simulink model "simpleInertiaModel"  (R2024a)
settings: Solver=ode23t  StartTime=0.0  StopTime=10  FixedStep=1e-3  MaxStep=0.01  RelTol=1e-3  AbsTol=1e-3  EnableMultiTasking=on
PreLoadFcn:
  | simpleInertiaModelParam
undefined symbols (not defined in the file): contact, objects, physics, ramp, X, Y, Z
libraries: sm_lib x47, fl_lib x33, nesl_utility x29
(part 1 of 2)
settings Model: Creator=lnicolet  LastModifiedBy=lnicolet
settings SolverCC: AutoScaleAbsTol=off  AlgebraicLoopSolver=TrustRegion  MaxZcPerStep=1
settings DataIOCC: LimitDataPoints=on  MaxDataPoints=10000  ReturnWorkspaceOutputsName=ssmInertia
settings OptimizationCC: ReuseModelBlockBuffer=off  LifeSpan=inf
settings DebuggingCC: UnconnectedInputMsg=warning  UnconnectedOutputMsg=warning  UnconnectedLineMsg=warning  AllowSymbolicDim=off  SubsystemReferenceDiagnosticForUnitTest=warning  SFUnexpectedBacktrackingDiag=warning  SFNoUnconditionalDefaultTransitionDiag=warning  SFExecutionAtInitializationDiag=none  ArithmeticOperatorsInVariantConditions=warning
settings ModelReferenceCC: EnableRefExpFcnMdlSchedulingChecks=on
settings SFSimCC: SimUseLocalCustomCode=off  CustomCodeUndefinedFunction=UseInterfaceOnly
settings RTWCC: RTWUseLocalCustomCode=off  GPUComputeCapability=3.5  DLArmComputeVersion=19.05
settings CodeAppCC: StateflowObjectComments=on
settings GRTTargetCC: TargetLangStandard=C89/C90 (ANSI)
settings ConfigComp: CovMetricSettings=dw  CovSaveCumulativeToWorkspaceVar=on  CovSaveSingleToWorkspaceVar=on  CovExternalEMLEnable=off  CovSFcnEnable=off
settings SimscapeCC: SimscapeLogType=all  SimscapeLogSimulationStatistics=on  SimscapeLogLimitData=off  SimscapeLogDataHistory=10000
settings ExplorerConfigSet: InternalSimMechanicsExplorerSettings="<ExplorerConfiguration><canonicalview>default</canonicalview><AnimationSetting><BasePlaybackSpeed>1.0</BasePlaybackSpeed><PlaybackSpeedFactor>1.0</PlaybackSpeedFactor></AnimationSetting><TilePanel><TileInfo><Tiles Columns=\"1\" Count=\"1\" Rows=\"1\"><Column Weight=\"1\"/><Row Weight=\"1\"/><Tile Height=\"1\" Width=\"1\" X=\"0\" Y=\"0\"/></Tiles></TileInfo><SceneInfo><SceneViewer><BGColor><R>0.60000002384185791</R><G>0.60000002384185791</G><B>0.60000002384185791</B></BGColor><Camera><DoPerspective>off</DoPerspective><Position><X>16.2073991208090149</X><Y>-6.20739939897376747</Y><Z>8.70739941654175098</Z></Position><Center><X>9.99999967767763209</X><Y>4.41576100129736915e-08</Y><Z>2.49999997341037261</Z></Center><Up><X>-0.408248290463863073</X><Y>0.408248290463863073</Y><Z>0.816496580927726145</Z></Up><ViewLimDist>1</ViewLimDist><YLim>7.56892333507537884</YLim><XLim>11.6046355697525012</XLim></Camera></SceneViewer></SceneInfo></TilePanel><MechEditorPanel><Cameras/><GfxPanelCameraMap/><VideoCreator><PlaybackSpeedRatio>1.0</PlaybackSpeedRatio><FrameRate>30</FrameRate><VideoFormat>Motion JPEG AVI</VideoFormat><FrameSize>auto</FrameSize></VideoCreator></MechEditorPanel></ExplorerConfiguration>"

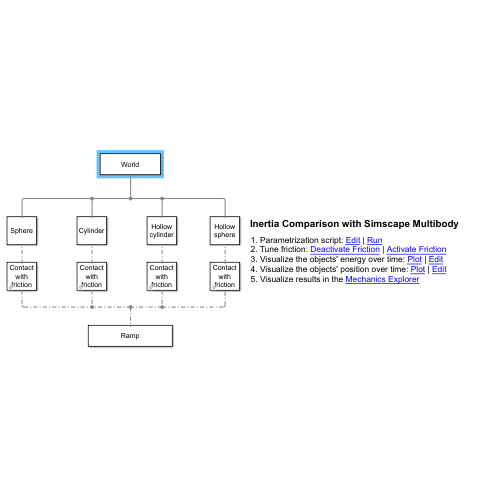
[thumbnail: Simulink's stored preview of the top-level diagram]
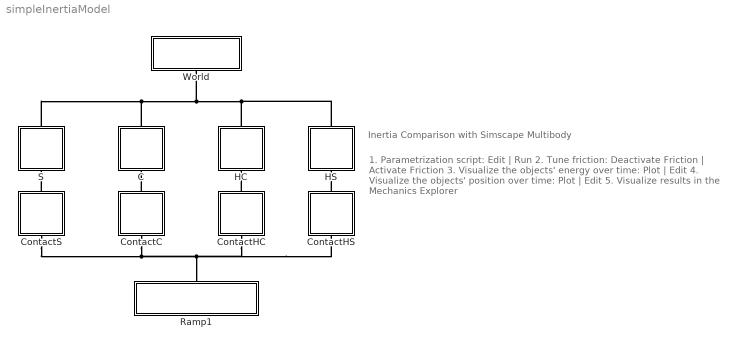
== system simpleInertiaModel ==
  note: 1. Parametrization script: Edit | Run
      | 2. Tune friction: Deactivate Friction | Activate Friction
      | 3. Visualize the objects' energy over time: Plot | Edit
      | 4. Visualize the objects' position over time: Plot | Edit
      | 5. Visualize results in the Mechanics Explorer
  note: Inertia Comparison with Simscape Multibody
  C : Subsystem
      mask Display: disp('Cylinder')
  ContactC : Subsystem  mask{c=contact.stiffness, d=contact.damping, tReg=contact.tansRegion, friction=Active, uS=contact.frictionStatic, uD=contact.frictionDynamic, v=contact.criticSpeed}
      mask prompts: c "Contact stiffness in N/m"; d "Contact damping in N/(m/s)"; tReg "Transition region in m"; friction "Contact Friction"; uS "Static friction coefficient"; uD "Dynamic friction coefficient"; v "Critical velocity in m/s"
      mask TypeOptions friction: Active | Inactive
      mask Callback friction:
      | ActiveChoice = get_param(gcb,'friction');
      | 
      |     switch ActiveChoice
      |         case 'Active'
      |             set_param([gcb,'/Ramp'],'FrictionType','SmoothStickSlip');
      |         case 'Inactive'
      |             set_param([gcb,'/Ramp'],'FrictionType','None');
      |     end
      mask DialogControl Container2 Prompt: Contact
      mask DialogControl Container3 Prompt: Friction
      mask Display:
      | ActiveChoice = get_param(gcb,'friction');
      | 
      | switch ActiveChoice
      |     case 'Active'
      |         disp('Contact\nwith\nfriction');
      |     case 'Inactive'
      |         disp('Contact\nwithout\nfriction');
      | end
  ContactHC : Subsystem  mask{c=contact.stiffness, d=contact.damping, tReg=contact.tansRegion, friction=Active, uS=contact.frictionStatic, uD=contact.frictionDynamic, v=contact.criticSpeed}
      mask prompts: c "Contact stiffness in N/m"; d "Contact damping in N/(m/s)"; tReg "Transition region in m"; friction "Contact Friction"; uS "Static friction coefficient"; uD "Dynamic friction coefficient"; v "Critical velocity in m/s"
      mask TypeOptions friction: Active | Inactive
      mask Callback friction:
      | ActiveChoice = get_param(gcb,'friction');
      | 
      |     switch ActiveChoice
      |         case 'Active'
      |             set_param([gcb,'/Ramp'],'FrictionType','SmoothStickSlip');
      |         case 'Inactive'
      |             set_param([gcb,'/Ramp'],'FrictionType','None');
      |     end
      mask DialogControl Container2 Prompt: Contact
      mask DialogControl Container3 Prompt: Friction
      mask Display:
      | ActiveChoice = get_param(gcb,'friction');
      | 
      | switch ActiveChoice
      |     case 'Active'
      |         disp('Contact\nwith\nfriction');
      |     case 'Inactive'
      |         disp('Contact\nwithout\nfriction');
      | end
  ContactHS : Subsystem  mask{c=contact.stiffness, d=contact.damping, tReg=contact.tansRegion, friction=Active, uS=contact.frictionStatic, uD=contact.frictionDynamic, v=contact.criticSpeed}
      mask prompts: c "Contact stiffness in N/m"; d "Contact damping in N/(m/s)"; tReg "Transition region in m"; friction "Contact Friction"; uS "Static friction coefficient"; uD "Dynamic friction coefficient"; v "Critical velocity in m/s"
      mask TypeOptions friction: Active | Inactive
      mask Callback friction:
      | ActiveChoice = get_param(gcb,'friction');
      | 
      |     switch ActiveChoice
      |         case 'Active'
      |             set_param([gcb,'/Ramp'],'FrictionType','SmoothStickSlip');
      |         case 'Inactive'
      |             set_param([gcb,'/Ramp'],'FrictionType','None');
      |     end
      mask DialogControl Container2 Prompt: Contact
      mask DialogControl Container3 Prompt: Friction
      mask Display:
      | ActiveChoice = get_param(gcb,'friction');
      | 
      | switch ActiveChoice
      |     case 'Active'
      |         disp('Contact\nwith\nfriction');
      |     case 'Inactive'
      |         disp('Contact\nwithout\nfriction');
      | end
  ContactS : Subsystem  mask{c=contact.stiffness, d=contact.damping, tReg=contact.tansRegion, friction=Active, uS=contact.frictionStatic, uD=contact.frictionDynamic, v=contact.criticSpeed}
      mask prompts: c "Contact stiffness in N/m"; d "Contact damping in N/(m/s)"; tReg "Transition region in m"; friction "Contact Friction"; uS "Static friction coefficient"; uD "Dynamic friction coefficient"; v "Critical velocity in m/s"
      mask TypeOptions friction: Active | Inactive
      mask Callback friction:
      | ActiveChoice = get_param(gcb,'friction');
      | 
      |     switch ActiveChoice
      |         case 'Active'
      |             set_param([gcb,'/Ramp'],'FrictionType','SmoothStickSlip');
      |         case 'Inactive'
      |             set_param([gcb,'/Ramp'],'FrictionType','None');
      |     end
      mask DialogControl Container2 Prompt: Contact
      mask DialogControl Container3 Prompt: Friction
      mask Display:
      | ActiveChoice = get_param(gcb,'friction');
      | 
      | switch ActiveChoice
      |     case 'Active'
      |         disp('Contact\nwith\nfriction');
      |     case 'Inactive'
      |         disp('Contact\nwithout\nfriction');
      | end
  HC : Subsystem
      mask Display: disp('Hollow\ncylinder')
  HS : Subsystem
      mask Display: disp('Hollow\nsphere')
  Ramp1 : Subsystem
      mask Display: disp('Ramp')
  S : Subsystem
      mask Display: disp('Sphere')
  World : Subsystem
      mask Display: disp('World')
  connections:
  C/LConn1 -- S/LConn1 -- HS/LConn1 -- HC/LConn1 -- World/RConn1
  ContactC/LConn1 -- C/RConn1
  ContactS/LConn1 -- S/RConn1
  ContactHS/LConn1 -- HS/RConn1
  ContactHC/LConn1 -- HC/RConn1
  ContactS/RConn1 -- ContactHS/RConn1 -- ContactHC/RConn1 -- Ramp1/LConn1 -- ContactC/RConn1

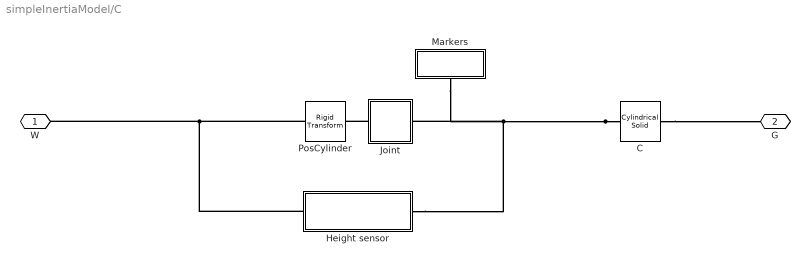
== system simpleInertiaModel/C ==
  C : sm_lib/Body Elements/Cylindrical Solid  CylinderRadius=objects.cylindRad  CylinderRadiusUnits=m  CylinderLength=objects.cylindLen  CylinderLengthUnits=m  ExportEntireGeometry=on  InertiaType=CalculateFromGeometry  BasedOnType=Mass  Density=cylindDen  DensityUnits=kg/m^3  Mass=physics.mass  MassUnits=kg  CenterOfMass=[0 0 0]  CenterOfMassUnits=m  MomentsOfInertia=[1 1 1]  MomentsOfInertiaUnits=kg*m^2  ProductsOfInertia=[0 0 0]  ProductsOfInertiaUnits=kg*m^2  GraphicType=FromGeometry  MarkerShape=Sphere  MarkerSize=10  GraphicVisPropType=SimpleVisualProperties  GraphicDiffuseColor=objects.cylindCol  GraphicOpacity=1  GraphicSpecularColor=[0.5 0.5 0.5 1.0]  GraphicAmbientColor=[0.15 0.15 0.15 1.0]  GraphicEmissiveColor=[0.0 0.0 0.0 1.0]  GraphicShininess=75  DoExposeReferenceFrame=off  SerializedFrames=<Frames><Frame><Id>Frame1</Id><Value><Name>F1</Name><Origin><Source>ReferenceFrame</Source><FeatureName></FeatureName></Origin><PrimaryAxis><DefinedDirection>+Y</DefinedDirection><Source>ReferenceFrame</Source><SourceDirection>+Z</SourceDirection><FeatureName></FeatureName></PrimaryAxis><SecondaryAxis><DefinedDirection>+X</DefinedDirection><Source>ReferenceFrame</Source><SourceDirection>+X</SourceDirection><FeatureName></FeatureName></SecondaryAxis></Value></Frame></Frames>
  Height sensor : Subsystem
      mask Display: disp('Height Sensor')
  Joint : Subsystem
      mask Display: disp('Joint')
  Markers : Subsystem
      mask Display: disp('Markers')
  PosCylinder : sm_lib/Frames and Transforms/Rigid Transform  RotationMethod=None  FollAlignAxisA=+X  BaseAlignAxisA=+Y  FollAlignAxisB=+Y  BaseAlignAxisB=+Z  RotationStandardAxis=+X  RotationAngle=90  RotationAngleUnits=deg  RotationArbitraryAxis=[0 0 1]  RotationSequenceAxes=FollowerAxes  RotationSequence=XYX  RotationSequenceAngles=[0 0 0]  RotationSequenceAnglesUnits=deg  RotationMatrix=[1 0 0; 0 1 0; 0 0 1]  Quaternion=[1 0 0 0]  TranslationMethod=Cartesian  TranslationCartesianOffset=objects.cylindPos  TranslationCartesianOffsetUnits=m  TranslationStandardAxis=+Z  TranslationStandardOffset=0  TranslationStandardOffsetUnits=m  TranslationROffset=0  TranslationROffsetUnits=m  TranslationThetaOffset=0  TranslationThetaOffsetUnits=deg  TranslationZOffset=0  TranslationZOffsetUnits=m
  W : PMIOPort  Side=Left
  G : PMIOPort  Port=2  Side=Right
  connections:
  C/RConn1 -- G/RConn1
  C/LConn1 -- Markers/LConn1 -- Joint/RConn1 -- Height sensor/RConn1
  PosCylinder/LConn1 -- Height sensor/LConn1 -- W/RConn1
  Joint/LConn1 -- PosCylinder/RConn1

== system simpleInertiaModel/ContactC ==
  Calculate Energies : Subsystem
  Ramp : sm_lib/Forces and Torques/Spatial Contact Force  NormalForceType=SmoothSpringDamper  NormalStiffness=c  NormalStiffnessUnits=N/m  NormalDamping=d  NormalDampingUnits=N/(m/s)  NormalTransitionRegionWidth=tReg  NormalTransitionRegionWidthUnits=m  FrictionType=SmoothStickSlip  CoefficientOfStaticFriction=uS  CoefficientOfDynamicFriction=uD  FrictionalCriticalVelocity=v  FrictionalCriticalVelocityUnits=m/s  SenseContactSignal=on  SensePenetrationDepth=on  SenseSeparationDistance=off  SenseNormalForceMagnitude=on  SenseFrictionalForceMagnitude=on  SenseNormalVelocity=on  SenseTangentialVelocity=on  SenseContactBaseRotation=off  SenseContactBaseTranslation=off  SenseContactFollowerRotation=off  SenseContactFollowerTranslation=off  ZeroCrossDetectContactStartAndEnd=off
  Terminator : Terminator
  CH : PMIOPort  Side=Left
  R1 : PMIOPort  Port=2  Side=Right
  wires:
  Calculate Energies/1(R) -> Terminator/1  "C"
  connections:
  Ramp/LConn1 -- CH/RConn1
  Ramp/RConn1 -- R1/RConn1
  Calculate Energies/LConn6 -- Ramp/RConn7
  Calculate Energies/LConn2 -- Ramp/RConn3
  Calculate Energies/LConn1 -- Ramp/RConn2
  Calculate Energies/LConn5 -- Ramp/RConn6
  Ramp/RConn5 -- Calculate Energies/LConn4
  Ramp/RConn4 -- Calculate Energies/LConn3

== system simpleInertiaModel/ContactHC ==
  Calculate Energies : Subsystem
  Ramp : sm_lib/Forces and Torques/Spatial Contact Force  NormalForceType=SmoothSpringDamper  NormalStiffness=c  NormalStiffnessUnits=N/m  NormalDamping=d  NormalDampingUnits=N/(m/s)  NormalTransitionRegionWidth=tReg  NormalTransitionRegionWidthUnits=m  FrictionType=SmoothStickSlip  CoefficientOfStaticFriction=uS  CoefficientOfDynamicFriction=uD  FrictionalCriticalVelocity=v  FrictionalCriticalVelocityUnits=m/s  SenseContactSignal=on  SensePenetrationDepth=on  SenseSeparationDistance=off  SenseNormalForceMagnitude=on  SenseFrictionalForceMagnitude=on  SenseNormalVelocity=on  SenseTangentialVelocity=on  SenseContactBaseRotation=off  SenseContactBaseTranslation=off  SenseContactFollowerRotation=off  SenseContactFollowerTranslation=off  ZeroCrossDetectContactStartAndEnd=off
  Terminator : Terminator
  CH : PMIOPort  Side=Left
  R1 : PMIOPort  Port=2  Side=Right
  wires:
  Calculate Energies/1(R) -> Terminator/1  "HC"
  connections:
  Ramp/LConn1 -- CH/RConn1
  Ramp/RConn1 -- R1/RConn1
  Ramp/RConn7 -- Calculate Energies/LConn6
  Ramp/RConn3 -- Calculate Energies/LConn2
  Ramp/RConn2 -- Calculate Energies/LConn1
  Ramp/RConn6 -- Calculate Energies/LConn5
  Ramp/RConn4 -- Calculate Energies/LConn3
  Ramp/RConn5 -- Calculate Energies/LConn4

== system simpleInertiaModel/ContactHS ==
  Calculate Energies : Subsystem
  Ramp : sm_lib/Forces and Torques/Spatial Contact Force  NormalForceType=SmoothSpringDamper  NormalStiffness=c  NormalStiffnessUnits=N/m  NormalDamping=d  NormalDampingUnits=N/(m/s)  NormalTransitionRegionWidth=tReg  NormalTransitionRegionWidthUnits=m  FrictionType=SmoothStickSlip  CoefficientOfStaticFriction=uS  CoefficientOfDynamicFriction=uD  FrictionalCriticalVelocity=v  FrictionalCriticalVelocityUnits=m/s  SenseContactSignal=on  SensePenetrationDepth=on  SenseSeparationDistance=off  SenseNormalForceMagnitude=on  SenseFrictionalForceMagnitude=on  SenseNormalVelocity=on  SenseTangentialVelocity=on  SenseContactBaseRotation=off  SenseContactBaseTranslation=off  SenseContactFollowerRotation=off  SenseContactFollowerTranslation=off  ZeroCrossDetectContactStartAndEnd=off
  Terminator : Terminator
  CH : PMIOPort  Side=Left
  R1 : PMIOPort  Port=2  Side=Right
  wires:
  Calculate Energies/1(R) -> Terminator/1  "HS"
  connections:
  Ramp/LConn1 -- CH/RConn1
  Ramp/RConn1 -- R1/RConn1
  Calculate Energies/LConn6 -- Ramp/RConn7
  Calculate Energies/LConn2 -- Ramp/RConn3
  Calculate Energies/LConn1 -- Ramp/RConn2
  Calculate Energies/LConn5 -- Ramp/RConn6
  Ramp/RConn5 -- Calculate Energies/LConn4
  Ramp/RConn4 -- Calculate Energies/LConn3

== system simpleInertiaModel/ContactS ==
  Calculate Energies : Subsystem
  Ramp : sm_lib/Forces and Torques/Spatial Contact Force  NormalForceType=SmoothSpringDamper  NormalStiffness=c  NormalStiffnessUnits=N/m  NormalDamping=d  NormalDampingUnits=N/(m/s)  NormalTransitionRegionWidth=tReg  NormalTransitionRegionWidthUnits=m  FrictionType=SmoothStickSlip  CoefficientOfStaticFriction=uS  CoefficientOfDynamicFriction=uD  FrictionalCriticalVelocity=v  FrictionalCriticalVelocityUnits=m/s  SenseContactSignal=on  SensePenetrationDepth=on  SenseSeparationDistance=off  SenseNormalForceMagnitude=on  SenseFrictionalForceMagnitude=on  SenseNormalVelocity=on  SenseTangentialVelocity=on  SenseContactBaseRotation=off  SenseContactBaseTranslation=off  SenseContactFollowerRotation=off  SenseContactFollowerTranslation=off  ZeroCrossDetectContactStartAndEnd=off
  Terminator : Terminator
  CH : PMIOPort  Side=Left
  R1 : PMIOPort  Port=2  Side=Right
  wires:
  Calculate Energies/1(R) -> Terminator/1  "S"
  connections:
  Ramp/LConn1 -- CH/RConn1
  Ramp/RConn1 -- R1/RConn1
  Calculate Energies/LConn6 -- Ramp/RConn7
  Calculate Energies/LConn2 -- Ramp/RConn3
  Calculate Energies/LConn1 -- Ramp/RConn2
  Calculate Energies/LConn5 -- Ramp/RConn6
  Ramp/RConn5 -- Calculate Energies/LConn4
  Ramp/RConn4 -- Calculate Energies/LConn3

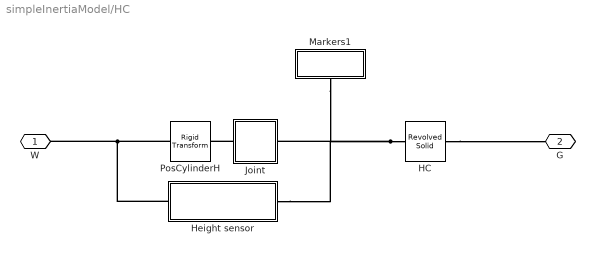
== system simpleInertiaModel/HC ==
  HC : sm_lib/Body Elements/Revolved Solid  RevolutionCrossSection=objects.cylindHPts  RevolutionCrossSectionUnits=m  RevolutionExtent=Full  RevolutionAngle=180  RevolutionAngleUnits=deg  ExportConvexHullGeometry=on  InertiaType=CalculateFromGeometry  BasedOnType=Mass  Density=1000  DensityUnits=kg/m^3  Mass=physics.mass  MassUnits=kg  CenterOfMass=[0 0 0]  CenterOfMassUnits=m  MomentsOfInertia=[1 1 1]  MomentsOfInertiaUnits=kg*m^2  ProductsOfInertia=[0 0 0]  ProductsOfInertiaUnits=kg*m^2  GraphicType=FromGeometry  MarkerShape=Sphere  MarkerSize=10  GraphicVisPropType=SimpleVisualProperties  GraphicDiffuseColor=objects.cylindHCol  GraphicOpacity=1  GraphicSpecularColor=[0.5 0.5 0.5 1.0]  GraphicAmbientColor=[0.15 0.15 0.15 1.0]  GraphicEmissiveColor=[0.0 0.0 0.0 1.0]  GraphicShininess=75  DoExposeReferenceFrame=off  SerializedFrames=<Frames><Frame><Id>Frame1</Id><Value><Name>F1</Name><Origin><Source>ReferenceFrame</Source><FeatureName></FeatureName></Origin><PrimaryAxis><DefinedDirection>+Y</DefinedDirection><Source>ReferenceFrame</Source><SourceDirection>+Z</SourceDirection><FeatureName></FeatureName></PrimaryAxis><SecondaryAxis><DefinedDirection>+X</DefinedDirection><Source>ReferenceFrame</Source><SourceDirection>+X</SourceDirection><FeatureName></FeatureName></SecondaryAxis></Value></Frame></Frames>
  Height sensor : Subsystem
      mask Display: disp('Height Sensor')
  Joint : Subsystem
      mask Display: disp('Joint')
  Markers1 : Subsystem
      mask Display: disp('Markers')
  PosCylinderH : sm_lib/Frames and Transforms/Rigid Transform  RotationMethod=None  FollAlignAxisA=+X  BaseAlignAxisA=+Y  FollAlignAxisB=+Y  BaseAlignAxisB=+Z  RotationStandardAxis=+X  RotationAngle=90  RotationAngleUnits=deg  RotationArbitraryAxis=[0 0 1]  RotationSequenceAxes=FollowerAxes  RotationSequence=XYX  RotationSequenceAngles=[0 0 0]  RotationSequenceAnglesUnits=deg  RotationMatrix=[1 0 0; 0 1 0; 0 0 1]  Quaternion=[1 0 0 0]  TranslationMethod=Cartesian  TranslationCartesianOffset=objects.cylindHPos  TranslationCartesianOffsetUnits=m  TranslationStandardAxis=+Z  TranslationStandardOffset=0  TranslationStandardOffsetUnits=m  TranslationROffset=0  TranslationROffsetUnits=m  TranslationThetaOffset=0  TranslationThetaOffsetUnits=deg  TranslationZOffset=0  TranslationZOffsetUnits=m
  W : PMIOPort  Side=Left
  G : PMIOPort  Port=2  Side=Right
  connections:
  PosCylinderH/LConn1 -- Height sensor/LConn1 -- W/RConn1
  HC/LConn1 -- Joint/RConn1 -- Height sensor/RConn1 -- Markers1/LConn1
  Joint/LConn1 -- PosCylinderH/RConn1
  HC/RConn1 -- G/RConn1

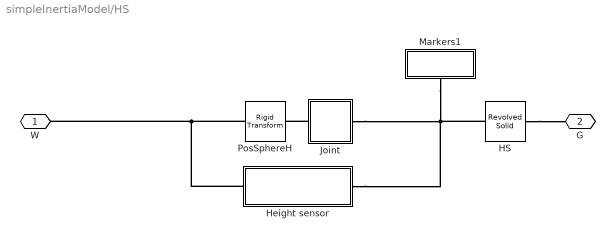
== system simpleInertiaModel/HS ==
  HS : sm_lib/Body Elements/Revolved Solid  RevolutionCrossSection=objects.sphereHPts  RevolutionCrossSectionUnits=m  RevolutionExtent=Full  RevolutionAngle=180  RevolutionAngleUnits=deg  ExportConvexHullGeometry=on  InertiaType=CalculateFromGeometry  BasedOnType=Mass  Density=1000  DensityUnits=kg/m^3  Mass=physics.mass  MassUnits=kg  CenterOfMass=[0 0 0]  CenterOfMassUnits=m  MomentsOfInertia=[1 1 1]  MomentsOfInertiaUnits=kg*m^2  ProductsOfInertia=[0 0 0]  ProductsOfInertiaUnits=kg*m^2  GraphicType=FromGeometry  MarkerShape=Sphere  MarkerSize=10  GraphicVisPropType=SimpleVisualProperties  GraphicDiffuseColor=objects.sphereHColor  GraphicOpacity=1  GraphicSpecularColor=[0.5 0.5 0.5 1.0]  GraphicAmbientColor=[0.15 0.15 0.15 1.0]  GraphicEmissiveColor=[0.0 0.0 0.0 1.0]  GraphicShininess=75  DoExposeReferenceFrame=on  SerializedFrames=<Frames/>
  Height sensor : Subsystem
      mask Display: disp('Height Sensor')
  Joint : Subsystem
      mask Display: disp('Joint')
  Markers1 : Subsystem
      mask Display: disp('Markers')
  PosSphereH : sm_lib/Frames and Transforms/Rigid Transform  RotationMethod=None  FollAlignAxisA=+X  BaseAlignAxisA=+Y  FollAlignAxisB=+Y  BaseAlignAxisB=+Z  RotationStandardAxis=+X  RotationAngle=90  RotationAngleUnits=deg  RotationArbitraryAxis=[0 0 1]  RotationSequenceAxes=FollowerAxes  RotationSequence=XYX  RotationSequenceAngles=[0 0 0]  RotationSequenceAnglesUnits=deg  RotationMatrix=[1 0 0; 0 1 0; 0 0 1]  Quaternion=[1 0 0 0]  TranslationMethod=Cartesian  TranslationCartesianOffset=objects.sphereHPos  TranslationCartesianOffsetUnits=m  TranslationStandardAxis=+Z  TranslationStandardOffset=0  TranslationStandardOffsetUnits=m  TranslationROffset=0  TranslationROffsetUnits=m  TranslationThetaOffset=0  TranslationThetaOffsetUnits=deg  TranslationZOffset=0  TranslationZOffsetUnits=m
  W : PMIOPort  Side=Left
  G : PMIOPort  Port=2  Side=Right
  connections:
  HS/LConn1 -- G/RConn1
  PosSphereH/LConn1 -- Height sensor/LConn1 -- W/RConn1
  Joint/RConn1 -- Height sensor/RConn1 -- Markers1/LConn1 -- HS/RConn1
  Joint/LConn1 -- PosSphereH/RConn1

== system simpleInertiaModel/Ramp1 ==
  PosRamp : sm_lib/Frames and Transforms/Rigid Transform  RotationMethod=StandardAxis  FollAlignAxisA=+X  BaseAlignAxisA=+Y  FollAlignAxisB=+Y  BaseAlignAxisB=+Z  RotationStandardAxis=+X  RotationAngle=90  RotationAngleUnits=deg  RotationArbitraryAxis=[0 0 1]  RotationSequenceAxes=FollowerAxes  RotationSequence=XYX  RotationSequenceAngles=[0 0 0]  RotationSequenceAnglesUnits=deg  RotationMatrix=[1 0 0; 0 1 0; 0 0 1]  Quaternion=[1 0 0 0]  TranslationMethod=None  TranslationCartesianOffset=[0 0 0]  TranslationCartesianOffsetUnits=m  TranslationStandardAxis=+Z  TranslationStandardOffset=0  TranslationStandardOffsetUnits=m  TranslationROffset=0  TranslationROffsetUnits=m  TranslationThetaOffset=0  TranslationThetaOffsetUnits=deg  TranslationZOffset=0  TranslationZOffsetUnits=m
  Ramp : sm_lib/Body Elements/Extruded Solid  ExtrusionType=General  PolygonNumSides=3  PolygonOuterRadius=1  PolygonOuterRadiusUnits=m  ExportEntireGeometry=off  ExtrusionCrossSection=ramp.rampPts  ExtrusionCrossSectionUnits=m  ExportConvexHullGeometry=on  ExtrusionLength=6  ExtrusionLengthUnits=m  InertiaType=CalculateFromGeometry  BasedOnType=Density  Density=1000  DensityUnits=kg/m^3  Mass=1  MassUnits=kg  CenterOfMass=[0 0 0]  CenterOfMassUnits=m  MomentsOfInertia=[1 1 1]  MomentsOfInertiaUnits=kg*m^2  ProductsOfInertia=[0 0 0]  ProductsOfInertiaUnits=kg*m^2  GraphicType=FromGeometry  MarkerShape=Sphere  MarkerSize=10  GraphicVisPropType=SimpleVisualProperties  GraphicDiffuseColor=[198,241,255]/255;  GraphicOpacity=1  GraphicSpecularColor=[0.5 0.5 0.5 1.0]  GraphicAmbientColor=[0.15 0.15 0.15 1.0]  GraphicEmissiveColor=[0.0 0.0 0.0 1.0]  GraphicShininess=75  DoExposeReferenceFrame=on  SerializedFrames=<Frames/>
  World Frame : sm_lib/Frames and Transforms/World Frame
  R1 : PMIOPort  Side=Left
  connections:
  Ramp/RConn1 -- PosRamp/RConn1
  Ramp/LConn1 -- R1/RConn1
  PosRamp/LConn1 -- World Frame/RConn1

== system simpleInertiaModel/S ==
  Height sensor : Subsystem
      mask Display: disp('Height Sensor')
  Joint : Subsystem
      mask Display: disp('Joint')
  Markers : Subsystem
      mask Display: disp('Markers')
  PosSphere : sm_lib/Frames and Transforms/Rigid Transform  RotationMethod=None  FollAlignAxisA=+X  BaseAlignAxisA=+Y  FollAlignAxisB=+Y  BaseAlignAxisB=+Z  RotationStandardAxis=+X  RotationAngle=90  RotationAngleUnits=deg  RotationArbitraryAxis=[0 0 1]  RotationSequenceAxes=FollowerAxes  RotationSequence=XYX  RotationSequenceAngles=[0 0 0]  RotationSequenceAnglesUnits=deg  RotationMatrix=[1 0 0; 0 1 0; 0 0 1]  Quaternion=[1 0 0 0]  TranslationMethod=Cartesian  TranslationCartesianOffset=objects.spherePos  TranslationCartesianOffsetUnits=m  TranslationStandardAxis=+Z  TranslationStandardOffset=0  TranslationStandardOffsetUnits=m  TranslationROffset=0  TranslationROffsetUnits=m  TranslationThetaOffset=0  TranslationThetaOffsetUnits=deg  TranslationZOffset=0  TranslationZOffsetUnits=m
  S : sm_lib/Body Elements/Spherical Solid  SphereRadius=objects.sphereRad  SphereRadiusUnits=m  ExportEntireGeometry=on  InertiaType=CalculateFromGeometry  BasedOnType=Mass  Density=1000  DensityUnits=kg/m^3  Mass=physics.mass  MassUnits=kg  CenterOfMass=[0 0 0]  CenterOfMassUnits=m  MomentsOfInertia=[1 1 1]  MomentsOfInertiaUnits=kg*m^2  ProductsOfInertia=[0 0 0]  ProductsOfInertiaUnits=kg*m^2  GraphicType=FromGeometry  MarkerShape=Sphere  MarkerSize=10  GraphicVisPropType=SimpleVisualProperties  GraphicDiffuseColor=objects.sphereColor  GraphicOpacity=1  GraphicSpecularColor=[0.5 0.5 0.5 1.0]  GraphicAmbientColor=[0.15 0.15 0.15 1.0]  GraphicEmissiveColor=[0.0 0.0 0.0 1.0]  GraphicShininess=75  DoExposeReferenceFrame=on  SerializedFrames=<Frames/>
  W : PMIOPort  Side=Left
  G : PMIOPort  Port=2  Side=Right
  connections:
  S/RConn1 -- Height sensor/RConn1 -- Joint/RConn1 -- Markers/LConn1
  PosSphere/RConn1 -- Joint/LConn1
  S/LConn1 -- G/RConn1
  W/RConn1 -- Height sensor/LConn1 -- PosSphere/LConn1

== system simpleInertiaModel/World ==
  Infinite Plane : sm_lib/Curves and Surfaces/Infinite Plane  GraphicType=Rectangle  GraphicPlaneWidth=ramp.rampLength+5  GraphicPlaneWidthUnits=m  GraphicPlaneHeight=12  GraphicPlaneHeightUnits=m  GraphicVisPropType=SimpleVisualProperties  GraphicDiffuseColor=[215,136,36]/255  GraphicOpacity=1  GraphicSpecularColor=[0.5 0.5 0.5 1.0]  GraphicAmbientColor=[0.15 0.15 0.15 1.0]  GraphicEmissiveColor=[0.0 0.0 0.0 1.0]  GraphicShininess=75
  Mechanism Configuration : sm_lib/Utilities/Mechanism Configuration  UniformGravity=Constant  GravityVector=[0 0 -physics.g]  GravityVectorUnits=m/s^2  LinearizationDelta=0.001  JointModeTransitionNonlinearIterations=2
  Rigid Transform : sm_lib/Frames and Transforms/Rigid Transform  RotationMethod=None  FollAlignAxisA=+X  BaseAlignAxisA=+Y  FollAlignAxisB=+Y  BaseAlignAxisB=+Z  RotationStandardAxis=+Z  RotationAngle=0  RotationAngleUnits=deg  RotationArbitraryAxis=[0 0 1]  RotationSequenceAxes=FollowerAxes  RotationSequence=XYX  RotationSequenceAngles=[0 0 0]  RotationSequenceAnglesUnits=deg  RotationMatrix=[1 0 0;0 1 0;0 0 1]  Quaternion=[1 0 0 0]  TranslationMethod=StandardAxis  TranslationCartesianOffset=[0 0 0]  TranslationCartesianOffsetUnits=m  TranslationStandardAxis=+X  TranslationStandardOffset=(ramp.rampLength+5)/2  TranslationStandardOffsetUnits=m  TranslationROffset=0  TranslationROffsetUnits=m  TranslationThetaOffset=0  TranslationThetaOffsetUnits=deg  TranslationZOffset=0  TranslationZOffsetUnits=m
  Solver Configuration : nesl_utility/Solver Configuration  PhysicalDomain=network_engine_domain  SubClassName=solver  LeftPortType=input  RightPortType=generic  Tones=[]  Harmonics=[]  SimulateNoise=off  Profile=off  UseLocalSampling=off  EnableSwitchedLinearOptims=on  FrequencyDomain=off  UseCCode=off  RelTol=0.001  AbsTol=1e-06  MinStep=1e-09  ToWorkspace=off  RevertToSquareIcSolve=off  NumHomotopyIterations=100  PhasorMode=off  PhasorModeNumHarmonics=1  ConsistencySolver=NEWTON_XTOL_AFTER_FTOL  IndexReductionMethod=DerivativeReplacement  DoDC=off  ResidualTolerance=1e-09  ConsistencyTolSource=GLOBAL  ConsistencyAbsTol=0.001  ConsistencyRelTol=0.001  ConsistencyTolFactor=0.001  UseLocalSolver=off  LocalSolverChoice=NE_BACKWARD_EULER_ADVANCER  ResolveIndetEquations=on  FunctionEvalNumThread=1  LocalSolverSampleTime=0.001  DoFixedCost=off  MaxNonlinIter=3  MaxModeIter=2  ComputeImpulses=off  ImpulseIterations=2  LinearAlgebra=Sparse  LinearAlgebraNumThread=0  EquationFormulation=NE_TIME_EF  DelaysMemoryBudget=1024  AutomaticFiltering=on  FilteringTimeConstant=0.001  PartitionStorageMethod=AS_NEEDED  PartitionMemoryBudget=1024  PartitionMethod=FAST  MultibodyUseLocalSolver=off  MultibodyLocalSolverChoice=ODE1  MultibodyLocalSolverSampleTime=0.001
  World Frame : sm_lib/Frames and Transforms/World Frame
  Conn3 : PMIOPort  Side=Right
  connections:
  Mechanism Configuration/RConn1 -- Rigid Transform/LConn1 -- World Frame/RConn1 -- Solver Configuration/RConn1 -- Conn3/RConn1
  Infinite Plane/LConn1 -- Rigid Transform/RConn1

== system simpleInertiaModel/C/Height sensor ==
  Simulation stopper : Subsystem
      mask Display: disp('Stop\n Simulation')
  Transform Sensor : sm_lib/Frames and Transforms/Transform Sensor  MeasurementFrame=World  RotationSequence=XYX  SenseAngle=off  SenseAxis=off  SenseQ=off  SenseR=off  SenseRotationSequence=off  SenseOmegaX=off  SenseOmegaY=off  SenseOmegaZ=off  SenseOmega=off  SenseQDot=off  SenseRDot=off  SenseRotationSequenceDot=off  SenseAlphaX=off  SenseAlphaY=off  SenseAlphaZ=off  SenseAlpha=off  SenseQDDot=off  SenseRDDot=off  SenseX=off  SenseY=off  SenseZ=on  SenseXYZ=off  SenseRad=off  SenseAzim=off  SenseDist=off  SenseInc=off  SenseXDot=off  SenseYDot=off  SenseZDot=off  SenseXYZDot=off  SenseRadDot=off  SenseAzimDot=off  SenseDistDot=off  SenseIncDot=off  SenseXDDot=off  SenseYDDot=off  SenseZDDot=off  SenseXYZDDot=off  SenseRadDDot=off  SenseAzimDDot=off  SenseDistDDot=off  SenseIncDDot=off
  pz : fl_lib/Physical Signals/Sinks/PS Terminator
  W : PMIOPort  Side=Left
  S : PMIOPort  Port=2  Side=Right
  connections:
  pz/LConn1 -- Transform Sensor/RConn2 -- Simulation stopper/LConn1
  Transform Sensor/LConn1 -- W/RConn1
  Transform Sensor/RConn1 -- S/RConn1

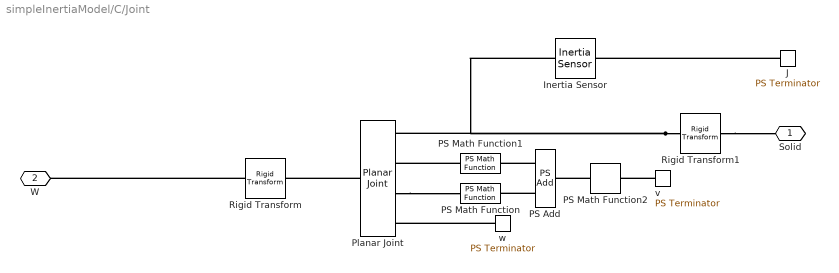
== system simpleInertiaModel/C/Joint ==
  Inertia Sensor : sm_lib/Body Elements/Inertia Sensor  SensorExtent=BodyGroup  SpanWeldJoints=off  ExcludeGroundedBodies=off  MeasurementFrame=World  SenseMass=off  SenseCenterOfMass=off  SenseInertiaMatrix=off  SenseCenteredInertiaMatrix=off  SensePrincipalInertiaMatrix=on  SenseRotationMatrix=off  GraphicType=None  PrincipalInertiaFrameSize=20  GraphicVisPropType=SimpleVisualProperties  GraphicDiffuseColor=[0.5 0.5 0.5]  GraphicOpacity=1  GraphicSpecularColor=[0.5 0.5 0.5 1.0]  GraphicAmbientColor=[0.15 0.15 0.15 1.0]  GraphicEmissiveColor=[0.0 0.0 0.0 1.0]  GraphicShininess=75
  J : fl_lib/Physical Signals/Sinks/PS Terminator
  PS Add : fl_lib/Physical Signals/Functions/PS Add
  PS Math Function : fl_lib/Physical Signals/Functions/PS Math Function  fcn_choice=foundation.enum.math_function.square  v=1
  PS Math Function1 : fl_lib/Physical Signals/Functions/PS Math Function  fcn_choice=foundation.enum.math_function.square  v=1
  PS Math Function2 : fl_lib/Physical Signals/Functions/PS Math Function  fcn_choice=foundation.enum.math_function.sqrt  v=1
  Planar Joint : sm_lib/Joints/Planar Joint  JointMode=Normal  CompositeWrenchDir=FollowerOnBase  CompositeWrenchFrame=BaseFrame  SenseConstraintForce=off  SenseConstraintTorque=off  SenseTotalForce=off  SenseTotalTorque=off  PxPositionTargetSpecify=off  PxPositionTargetPriority=High  PxPositionTargetValue=0  PxPositionTargetValueUnits=m  PxVelocityTargetSpecify=off  PxVelocityTargetPriority=High  PxVelocityTargetValue=0  PxVelocityTargetValueUnits=m/s  PxEquilibriumPosition=0  PxEquilibriumPositionUnits=m  PxSpringStiffness=0  PxSpringStiffnessUnits=N/m  PxDampingCoefficient=0  PxDampingCoefficientUnits=N/(m/s)  PxLowerLimitSpecify=off  PxLowerLimitBound=-1  PxLowerLimitBoundUnits=m  PxLowerLimitStiffness=1e6  PxLowerLimitStiffnessUnits=N/m  PxLowerLimitDamping=1e3  PxLowerLimitDampingUnits=N/(m/s)  PxLowerLimitTransitionRegionWidth=1e-4  PxLowerLimitTransitionRegionWidthUnits=m  PxUpperLimitSpecify=off  PxUpperLimitBound=1  PxUpperLimitBoundUnits=m  PxUpperLimitStiffness=1e6  PxUpperLimitStiffnessUnits=N/m  PxUpperLimitDamping=1e3  PxUpperLimitDampingUnits=N/(m/s)  PxUpperLimitTransitionRegionWidth=1e-4  PxUpperLimitTransitionRegionWidthUnits=m  PxTorqueActuationMode=NoTorque  PxMotionActuationMode=ComputedMotion  PxSensePosition=off  PxSenseVelocity=on  PxSenseAcceleration=off  PxSenseTorqueForce=off  PxSenseLowerLimitTorqueForce=off  PxSenseUpperLimitTorqueForce=off  PyPositionTargetSpecify=off  PyPositionTargetPriority=High  PyPositionTargetValue=0  PyPositionTargetValueUnits=m  PyVelocityTargetSpecify=off  PyVelocityTargetPriority=High  PyVelocityTargetValue=0  PyVelocityTargetValueUnits=m/s  PyEquilibriumPosition=0  PyEquilibriumPositionUnits=m  PySpringStiffness=0  PySpringStiffnessUnits=N/m  PyDampingCoefficient=0  PyDampingCoefficientUnits=N/(m/s)  PyLowerLimitSpecify=off  PyLowerLimitBound=-1  PyLowerLimitBoundUnits=m  PyLowerLimitStiffness=1e6  PyLowerLimitStiffnessUnits=N/m  PyLowerLimitDamping=1e3  PyLowerLimitDampingUnits=N/(m/s)  PyLowerLimitTransitionRegionWidth=1e-4  PyLowerLimitTransitionRegionWidthUnits=m  PyUpperLimitSpecify=off  PyUpperLimitBound=1  PyUpperLimitBoundUnits=m  PyUpperLimitStiffness=1e6  PyUpperLimitStiffnessUnits=N/m  PyUpperLimitDamping=1e3  PyUpperLimitDampingUnits=N/(m/s)  PyUpperLimitTransitionRegionWidth=1e-4  PyUpperLimitTransitionRegionWidthUnits=m  PyTorqueActuationMode=NoTorque  PyMotionActuationMode=ComputedMotion  PySensePosition=off  PySenseVelocity=on  PySenseAcceleration=off  PySenseTorqueForce=off  PySenseLowerLimitTorqueForce=off  PySenseUpperLimitTorqueForce=off  RzPositionTargetSpecify=off  RzPositionTargetPriority=High  RzPositionTargetValue=0  RzPositionTargetValueUnits=deg  RzVelocityTargetSpecify=off  RzVelocityTargetPriority=High  RzVelocityTargetValue=0  RzVelocityTargetValueUnits=deg/s  RzEquilibriumPosition=0  RzEquilibriumPositionUnits=deg  RzSpringStiffness=0  RzSpringStiffnessUnits=N*m/deg  RzDampingCoefficient=0  RzDampingCoefficientUnits=N*m/(deg/s)  RzLowerLimitSpecify=off  RzLowerLimitBound=-90  RzLowerLimitBoundUnits=deg  RzLowerLimitStiffness=1e4  RzLowerLimitStiffnessUnits=N*m/deg  RzLowerLimitDamping=10  RzLowerLimitDampingUnits=N*m/(deg/s)  RzLowerLimitTransitionRegionWidth=0.1  RzLowerLimitTransitionRegionWidthUnits=deg  RzUpperLimitSpecify=off  RzUpperLimitBound=90  RzUpperLimitBoundUnits=deg  RzUpperLimitStiffness=1e4  RzUpperLimitStiffnessUnits=N*m/deg  RzUpperLimitDamping=10  RzUpperLimitDampingUnits=N*m/(deg/s)  RzUpperLimitTransitionRegionWidth=0.1  RzUpperLimitTransitionRegionWidthUnits=deg  RzTorqueActuationMode=NoTorque  RzMotionActuationMode=ComputedMotion  RzSensePosition=off  RzSenseVelocity=on  RzSenseAcceleration=off  RzSenseTorqueForce=off  RzSenseLowerLimitTorqueForce=off  RzSenseUpperLimitTorqueForce=off
  Rigid Transform : sm_lib/Frames and Transforms/Rigid Transform  RotationMethod=StandardAxis  FollAlignAxisA=+X  BaseAlignAxisA=+Y  FollAlignAxisB=+Y  BaseAlignAxisB=+Z  RotationStandardAxis=+X  RotationAngle=90  RotationAngleUnits=deg  RotationArbitraryAxis=[0 0 1]  RotationSequenceAxes=FollowerAxes  RotationSequence=XYX  RotationSequenceAngles=[0 0 0]  RotationSequenceAnglesUnits=deg  RotationMatrix=[1 0 0;0 1 0;0 0 1]  Quaternion=[1 0 0 0]  TranslationMethod=None  TranslationCartesianOffset=[0 0 0]  TranslationCartesianOffsetUnits=m  TranslationStandardAxis=+Z  TranslationStandardOffset=0  TranslationStandardOffsetUnits=m  TranslationROffset=0  TranslationROffsetUnits=m  TranslationThetaOffset=0  TranslationThetaOffsetUnits=deg  TranslationZOffset=0  TranslationZOffsetUnits=m
  Rigid Transform1 : sm_lib/Frames and Transforms/Rigid Transform  RotationMethod=StandardAxis  FollAlignAxisA=+X  BaseAlignAxisA=+Y  FollAlignAxisB=+Y  BaseAlignAxisB=+Z  RotationStandardAxis=+X  RotationAngle=-90  RotationAngleUnits=deg  RotationArbitraryAxis=[0 0 1]  RotationSequenceAxes=FollowerAxes  RotationSequence=XYX  RotationSequenceAngles=[0 0 0]  RotationSequenceAnglesUnits=deg  RotationMatrix=[1 0 0;0 1 0;0 0 1]  Quaternion=[1 0 0 0]  TranslationMethod=None  TranslationCartesianOffset=[0 0 0]  TranslationCartesianOffsetUnits=m  TranslationStandardAxis=+Z  TranslationStandardOffset=0  TranslationStandardOffsetUnits=m  TranslationROffset=0  TranslationROffsetUnits=m  TranslationThetaOffset=0  TranslationThetaOffsetUnits=deg  TranslationZOffset=0  TranslationZOffsetUnits=m
  v : fl_lib/Physical Signals/Sinks/PS Terminator
  w : fl_lib/Physical Signals/Sinks/PS Terminator
  Solid : PMIOPort  Side=Right
  W : PMIOPort  Port=2  Side=Left
  connections:
  Rigid Transform1/LConn1 -- Inertia Sensor/LConn1 -- Planar Joint/RConn1
  Rigid Transform/LConn1 -- W/RConn1
  Rigid Transform1/RConn1 -- Solid/RConn1
  w/LConn1 -- Planar Joint/RConn4
  J/LConn1 -- Inertia Sensor/RConn1
  Planar Joint/LConn1 -- Rigid Transform/RConn1
  PS Math Function1/LConn1 -- Planar Joint/RConn2
  v/LConn1 -- PS Math Function2/RConn1
  PS Add/LConn1 -- PS Math Function1/RConn1
  PS Math Function2/LConn1 -- PS Add/RConn1
  PS Add/LConn2 -- PS Math Function/RConn1
  Planar Joint/RConn3 -- PS Math Function/LConn1

== system simpleInertiaModel/C/Markers ==
  Extruded Solid2 : sm_lib/Body Elements/Extruded Solid  ExtrusionType=General  PolygonNumSides=3  PolygonOuterRadius=1  PolygonOuterRadiusUnits=m  ExportEntireGeometry=off  ExtrusionCrossSection=objects.markerCPts  ExtrusionCrossSectionUnits=m  ExportConvexHullGeometry=off  ExtrusionLength=0.1  ExtrusionLengthUnits=m  InertiaType=CalculateFromGeometry  BasedOnType=Density  Density=0  DensityUnits=kg/m^3  Mass=1  MassUnits=kg  CenterOfMass=[0 0 0]  CenterOfMassUnits=m  MomentsOfInertia=[1 1 1]  MomentsOfInertiaUnits=kg*m^2  ProductsOfInertia=[0 0 0]  ProductsOfInertiaUnits=kg*m^2  GraphicType=FromGeometry  MarkerShape=Sphere  MarkerSize=10  GraphicVisPropType=SimpleVisualProperties  GraphicDiffuseColor=[1.0 0.0 0.2]  GraphicOpacity=1  GraphicSpecularColor=[0.5 0.5 0.5 1.0]  GraphicAmbientColor=[0.15 0.15 0.15 1.0]  GraphicEmissiveColor=[0.0 0.0 0.0 1.0]  GraphicShininess=75  DoExposeReferenceFrame=off  SerializedFrames=<Frames><Frame><Id>Frame1</Id><Value><Name>F1</Name><Origin><Source>ReferenceFrame</Source><FeatureName></FeatureName></Origin><PrimaryAxis><DefinedDirection>-Y</DefinedDirection><Source>ReferenceFrame</Source><SourceDirection>+Z</SourceDirection><FeatureName></FeatureName></PrimaryAxis><SecondaryAxis><DefinedDirection>-Z</DefinedDirection><Source>ReferenceFrame</Source><SourceDirection>+X</SourceDirection><FeatureName></FeatureName></SecondaryAxis></Value></Frame></Frames>
  Extruded Solid3 : sm_lib/Body Elements/Extruded Solid  ExtrusionType=General  PolygonNumSides=3  PolygonOuterRadius=1  PolygonOuterRadiusUnits=m  ExportEntireGeometry=off  ExtrusionCrossSection=objects.markerCPts  ExtrusionCrossSectionUnits=m  ExportConvexHullGeometry=off  ExtrusionLength=0.1  ExtrusionLengthUnits=m  InertiaType=CalculateFromGeometry  BasedOnType=Density  Density=0  DensityUnits=kg/m^3  Mass=1  MassUnits=kg  CenterOfMass=[0 0 0]  CenterOfMassUnits=m  MomentsOfInertia=[1 1 1]  MomentsOfInertiaUnits=kg*m^2  ProductsOfInertia=[0 0 0]  ProductsOfInertiaUnits=kg*m^2  GraphicType=FromGeometry  MarkerShape=Sphere  MarkerSize=10  GraphicVisPropType=SimpleVisualProperties  GraphicDiffuseColor=[1.0 0.0 0.2]  GraphicOpacity=1  GraphicSpecularColor=[0.5 0.5 0.5 1.0]  GraphicAmbientColor=[0.15 0.15 0.15 1.0]  GraphicEmissiveColor=[0.0 0.0 0.0 1.0]  GraphicShininess=75  DoExposeReferenceFrame=off  SerializedFrames=<Frames><Frame><Id>Frame1</Id><Value><Name>F1</Name><Origin><Source>ReferenceFrame</Source><FeatureName></FeatureName></Origin><PrimaryAxis><DefinedDirection>-Y</DefinedDirection><Source>ReferenceFrame</Source><SourceDirection>+Z</SourceDirection><FeatureName></FeatureName></PrimaryAxis><SecondaryAxis><DefinedDirection>+Z</DefinedDirection><Source>ReferenceFrame</Source><SourceDirection>+X</SourceDirection><FeatureName></FeatureName></SecondaryAxis></Value></Frame></Frames>
  Conn1 : PMIOPort  Side=Left
  connections:
  Extruded Solid3/LConn1 -- Extruded Solid2/LConn1 -- Conn1/RConn1

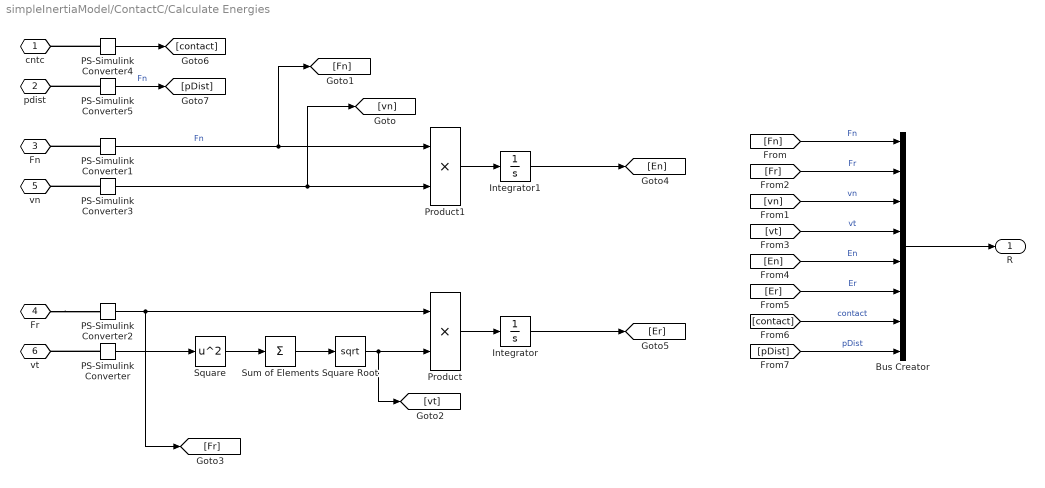
== system simpleInertiaModel/ContactC/Calculate Energies ==
  Bus Creator : BusCreator  Inputs=8
  Integrator : Integrator
  Integrator1 : Integrator
  PS-Simulink Converter : nesl_utility/PS-Simulink Converter  PhysicalDomain=network_engine_domain  SubClassName=ps_output  LeftPortType=input  RightPortType=output  PseudoPeriodic=off  Frequencies=[]  VectorFormat=inherit  Unit=m/s  AffineConversion=off
  PS-Simulink Converter1 : nesl_utility/PS-Simulink Converter  PhysicalDomain=network_engine_domain  SubClassName=ps_output  LeftPortType=input  RightPortType=output  PseudoPeriodic=off  Frequencies=[]  VectorFormat=inherit  Unit=N  AffineConversion=off
  PS-Simulink Converter2 : nesl_utility/PS-Simulink Converter  PhysicalDomain=network_engine_domain  SubClassName=ps_output  LeftPortType=input  RightPortType=output  PseudoPeriodic=off  Frequencies=[]  VectorFormat=inherit  Unit=N  AffineConversion=off
  PS-Simulink Converter3 : nesl_utility/PS-Simulink Converter  PhysicalDomain=network_engine_domain  SubClassName=ps_output  LeftPortType=input  RightPortType=output  PseudoPeriodic=off  Frequencies=[]  VectorFormat=inherit  Unit=m/s  AffineConversion=off
  PS-Simulink Converter4 : nesl_utility/PS-Simulink Converter  PhysicalDomain=network_engine_domain  SubClassName=ps_output  LeftPortType=input  RightPortType=output  PseudoPeriodic=off  Frequencies=[]  VectorFormat=inherit  Unit=mm  AffineConversion=off
  PS-Simulink Converter5 : nesl_utility/PS-Simulink Converter  PhysicalDomain=network_engine_domain  SubClassName=ps_output  LeftPortType=input  RightPortType=output  PseudoPeriodic=off  Frequencies=[]  VectorFormat=inherit  Unit=mm  AffineConversion=off
  Product : Product
  Product1 : Product
  Square : Math  Operator=square
  Square Root : Sqrt
  Sum of Elements : Sum  Inputs=+
  cntc : PMIOPort  Side=Left
  pdist : PMIOPort  Port=2  Side=Left
  Fn : PMIOPort  Port=3  Side=Left
  Fr : PMIOPort  Port=4  Side=Left
  vn : PMIOPort  Port=5  Side=Left
  vt : PMIOPort  Port=6  Side=Left
  R : Outport
  wires:
  Bus Creator/1 -> R/1
  [Er] -> Bus Creator/6  "Er"
  [En] -> Bus Creator/5  "En"
  [vt] -> Bus Creator/4  "vt"
  [Fr] -> Bus Creator/2  "Fr"
  [vn] -> Bus Creator/3  "vn"
  [Fn] -> Bus Creator/1  "Fn"
  Integrator/1 -> [Er]
  Integrator1/1 -> [En]
  PS-Simulink Converter3/1 -> Product1/2, [vn]
  Product1/1 -> Integrator1/1
  PS-Simulink Converter1/1 -> Product1/1, [Fn]  "Fn"
  Product/1 -> Integrator/1
  Square Root/1 -> [vt], Product/2
  Square/1 -> Sum of Elements/1
  PS-Simulink Converter/1 -> Square/1
  Sum of Elements/1 -> Square Root/1
  PS-Simulink Converter4/1 -> [contact]
  PS-Simulink Converter5/1 -> [pDist]  "Fn"
  [contact] -> Bus Creator/7  "contact"
  [pDist] -> Bus Creator/8  "pDist"
  PS-Simulink Converter2/1 -> Product/1, [Fr]
  connections:
  PS-Simulink Converter3/LConn1 -- vn/RConn1
  Fr/RConn1 -- PS-Simulink Converter2/LConn1
  PS-Simulink Converter1/LConn1 -- Fn/RConn1
  PS-Simulink Converter/LConn1 -- vt/RConn1
  PS-Simulink Converter4/LConn1 -- cntc/RConn1
  PS-Simulink Converter5/LConn1 -- pdist/RConn1

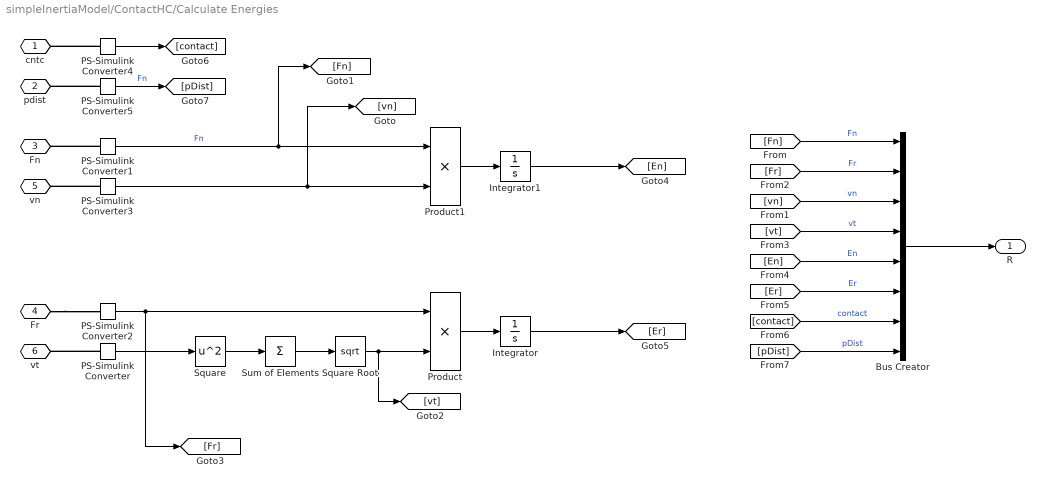
== system simpleInertiaModel/ContactHC/Calculate Energies ==
  Bus Creator : BusCreator  Inputs=8
  Integrator : Integrator
  Integrator1 : Integrator
  PS-Simulink Converter : nesl_utility/PS-Simulink Converter  PhysicalDomain=network_engine_domain  SubClassName=ps_output  LeftPortType=input  RightPortType=output  PseudoPeriodic=off  Frequencies=[]  VectorFormat=inherit  Unit=m/s  AffineConversion=off
  PS-Simulink Converter1 : nesl_utility/PS-Simulink Converter  PhysicalDomain=network_engine_domain  SubClassName=ps_output  LeftPortType=input  RightPortType=output  PseudoPeriodic=off  Frequencies=[]  VectorFormat=inherit  Unit=N  AffineConversion=off
  PS-Simulink Converter2 : nesl_utility/PS-Simulink Converter  PhysicalDomain=network_engine_domain  SubClassName=ps_output  LeftPortType=input  RightPortType=output  PseudoPeriodic=off  Frequencies=[]  VectorFormat=inherit  Unit=N  AffineConversion=off
  PS-Simulink Converter3 : nesl_utility/PS-Simulink Converter  PhysicalDomain=network_engine_domain  SubClassName=ps_output  LeftPortType=input  RightPortType=output  PseudoPeriodic=off  Frequencies=[]  VectorFormat=inherit  Unit=m/s  AffineConversion=off
  PS-Simulink Converter4 : nesl_utility/PS-Simulink Converter  PhysicalDomain=network_engine_domain  SubClassName=ps_output  LeftPortType=input  RightPortType=output  PseudoPeriodic=off  Frequencies=[]  VectorFormat=inherit  Unit=mm  AffineConversion=off
  PS-Simulink Converter5 : nesl_utility/PS-Simulink Converter  PhysicalDomain=network_engine_domain  SubClassName=ps_output  LeftPortType=input  RightPortType=output  PseudoPeriodic=off  Frequencies=[]  VectorFormat=inherit  Unit=mm  AffineConversion=off
  Product : Product
  Product1 : Product
  Square : Math  Operator=square
  Square Root : Sqrt
  Sum of Elements : Sum  Inputs=+
  cntc : PMIOPort  Side=Left
  pdist : PMIOPort  Port=2  Side=Left
  Fn : PMIOPort  Port=3  Side=Left
  Fr : PMIOPort  Port=4  Side=Left
  vn : PMIOPort  Port=5  Side=Left
  vt : PMIOPort  Port=6  Side=Left
  R : Outport
  wires:
  Bus Creator/1 -> R/1
  [Er] -> Bus Creator/6  "Er"
  [En] -> Bus Creator/5  "En"
  [vt] -> Bus Creator/4  "vt"
  [Fr] -> Bus Creator/2  "Fr"
  [vn] -> Bus Creator/3  "vn"
  [Fn] -> Bus Creator/1  "Fn"
  Integrator/1 -> [Er]
  Integrator1/1 -> [En]
  PS-Simulink Converter3/1 -> Product1/2, [vn]
  Product1/1 -> Integrator1/1
  PS-Simulink Converter1/1 -> Product1/1, [Fn]  "Fn"
  Product/1 -> Integrator/1
  Square Root/1 -> [vt], Product/2
  Square/1 -> Sum of Elements/1
  PS-Simulink Converter/1 -> Square/1
  Sum of Elements/1 -> Square Root/1
  PS-Simulink Converter4/1 -> [contact]
  PS-Simulink Converter5/1 -> [pDist]  "Fn"
  [contact] -> Bus Creator/7  "contact"
  [pDist] -> Bus Creator/8  "pDist"
  PS-Simulink Converter2/1 -> Product/1, [Fr]
  connections:
  PS-Simulink Converter3/LConn1 -- vn/RConn1
  Fr/RConn1 -- PS-Simulink Converter2/LConn1
  PS-Simulink Converter1/LConn1 -- Fn/RConn1
  PS-Simulink Converter/LConn1 -- vt/RConn1
  PS-Simulink Converter4/LConn1 -- cntc/RConn1
  PS-Simulink Converter5/LConn1 -- pdist/RConn1

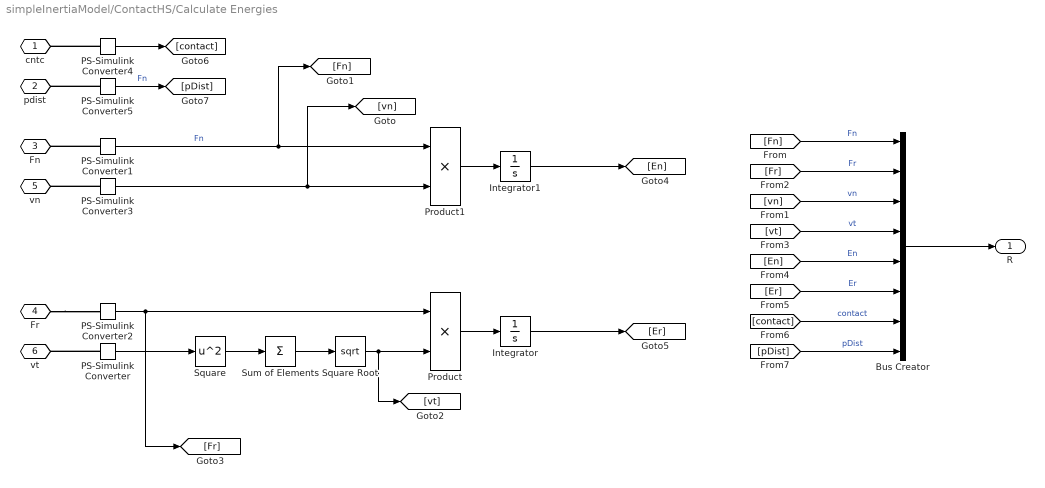
== system simpleInertiaModel/ContactHS/Calculate Energies ==
  Bus Creator : BusCreator  Inputs=8
  Integrator : Integrator
  Integrator1 : Integrator
  PS-Simulink Converter : nesl_utility/PS-Simulink Converter  PhysicalDomain=network_engine_domain  SubClassName=ps_output  LeftPortType=input  RightPortType=output  PseudoPeriodic=off  Frequencies=[]  VectorFormat=inherit  Unit=m/s  AffineConversion=off
  PS-Simulink Converter1 : nesl_utility/PS-Simulink Converter  PhysicalDomain=network_engine_domain  SubClassName=ps_output  LeftPortType=input  RightPortType=output  PseudoPeriodic=off  Frequencies=[]  VectorFormat=inherit  Unit=N  AffineConversion=off
  PS-Simulink Converter2 : nesl_utility/PS-Simulink Converter  PhysicalDomain=network_engine_domain  SubClassName=ps_output  LeftPortType=input  RightPortType=output  PseudoPeriodic=off  Frequencies=[]  VectorFormat=inherit  Unit=N  AffineConversion=off
  PS-Simulink Converter3 : nesl_utility/PS-Simulink Converter  PhysicalDomain=network_engine_domain  SubClassName=ps_output  LeftPortType=input  RightPortType=output  PseudoPeriodic=off  Frequencies=[]  VectorFormat=inherit  Unit=m/s  AffineConversion=off
  PS-Simulink Converter4 : nesl_utility/PS-Simulink Converter  PhysicalDomain=network_engine_domain  SubClassName=ps_output  LeftPortType=input  RightPortType=output  PseudoPeriodic=off  Frequencies=[]  VectorFormat=inherit  Unit=mm  AffineConversion=off
  PS-Simulink Converter5 : nesl_utility/PS-Simulink Converter  PhysicalDomain=network_engine_domain  SubClassName=ps_output  LeftPortType=input  RightPortType=output  PseudoPeriodic=off  Frequencies=[]  VectorFormat=inherit  Unit=mm  AffineConversion=off
  Product : Product
  Product1 : Product
  Square : Math  Operator=square
  Square Root : Sqrt
  Sum of Elements : Sum  Inputs=+
  cntc : PMIOPort  Side=Left
  pdist : PMIOPort  Port=2  Side=Left
  Fn : PMIOPort  Port=3  Side=Left
  Fr : PMIOPort  Port=4  Side=Left
  vn : PMIOPort  Port=5  Side=Left
  vt : PMIOPort  Port=6  Side=Left
  R : Outport
  wires:
  Bus Creator/1 -> R/1
  [Er] -> Bus Creator/6  "Er"
  [En] -> Bus Creator/5  "En"
  [vt] -> Bus Creator/4  "vt"
  [Fr] -> Bus Creator/2  "Fr"
  [vn] -> Bus Creator/3  "vn"
  [Fn] -> Bus Creator/1  "Fn"
  Integrator/1 -> [Er]
  Integrator1/1 -> [En]
  PS-Simulink Converter3/1 -> Product1/2, [vn]
  Product1/1 -> Integrator1/1
  PS-Simulink Converter1/1 -> Product1/1, [Fn]  "Fn"
  Product/1 -> Integrator/1
  Square Root/1 -> [vt], Product/2
  Square/1 -> Sum of Elements/1
  PS-Simulink Converter/1 -> Square/1
  Sum of Elements/1 -> Square Root/1
  PS-Simulink Converter4/1 -> [contact]
  PS-Simulink Converter5/1 -> [pDist]  "Fn"
  [contact] -> Bus Creator/7  "contact"
  [pDist] -> Bus Creator/8  "pDist"
  PS-Simulink Converter2/1 -> Product/1, [Fr]
  connections:
  PS-Simulink Converter3/LConn1 -- vn/RConn1
  Fr/RConn1 -- PS-Simulink Converter2/LConn1
  PS-Simulink Converter1/LConn1 -- Fn/RConn1
  PS-Simulink Converter/LConn1 -- vt/RConn1
  PS-Simulink Converter4/LConn1 -- cntc/RConn1
  PS-Simulink Converter5/LConn1 -- pdist/RConn1
